simulink model "Catwell_Rom"  (R2023b)
settings: Solver=FixedStepDiscrete  StartTime=0.0  StopTime=3.999  FixedStep=0.02  RelTol=1e-3
libraries: Pathfinding_lib x2, drivinglib x1, SignalEditorBlockLib x1, matrix_library x1
settings Model: Creator=FIRSTMentor  LastModifiedBy=FIRSTMentor
settings OptimizationCC: DefaultParameterBehavior=Inlined  EnhancedBackFolding=on  PassReuseOutputArgsAs=Individual arguments  ZeroExternalMemoryAtStartup=off  ZeroInternalMemoryAtStartup=off  OptimizeBlockOrder=speed  DifferentSizesBufferReuse=on  OptimizationCustomize=off  EfficientTunableParamExpr=on
settings DebuggingCC: ParameterTunabilityLossMsg=error
settings SFSimCC: MATLABDynamicMemAlloc=off
settings RTWCC: Description=Embedded Coder  SystemTargetFile=ert.tlc  GenCodeOnly=on  TemplateMakefile=ert_default_tmf  Toolchain=Microsoft Visual C++ 2022 v17.0 | CMake/nmake (64-bit Windows)  BuildConfiguration=Release
settings CodeAppCC: ForceParamTrailComments=on  IgnoreCustomStorageClasses=off  OperatorAnnotations=on  SimulinkDataObjDesc=on  SFDataObjDesc=on  InsertBlockDesc=on
settings ERTTargetCC: TargetLangStandard=C99 (ISO)  GenerateSampleERTMain=on  InlinedParameterPlacement=NonHierarchical  ERTCustomFileTemplate=example_file_process.tlc

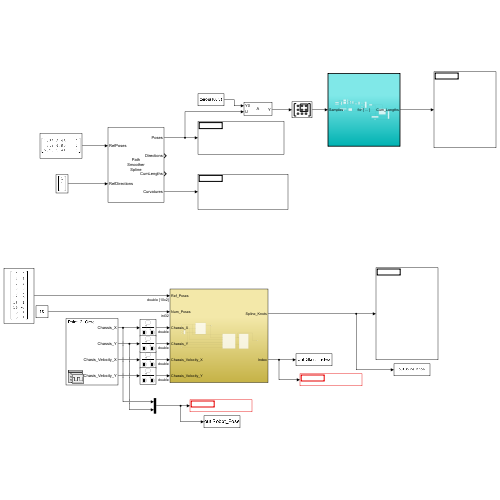
[thumbnail: Simulink's stored preview of the top-level diagram]
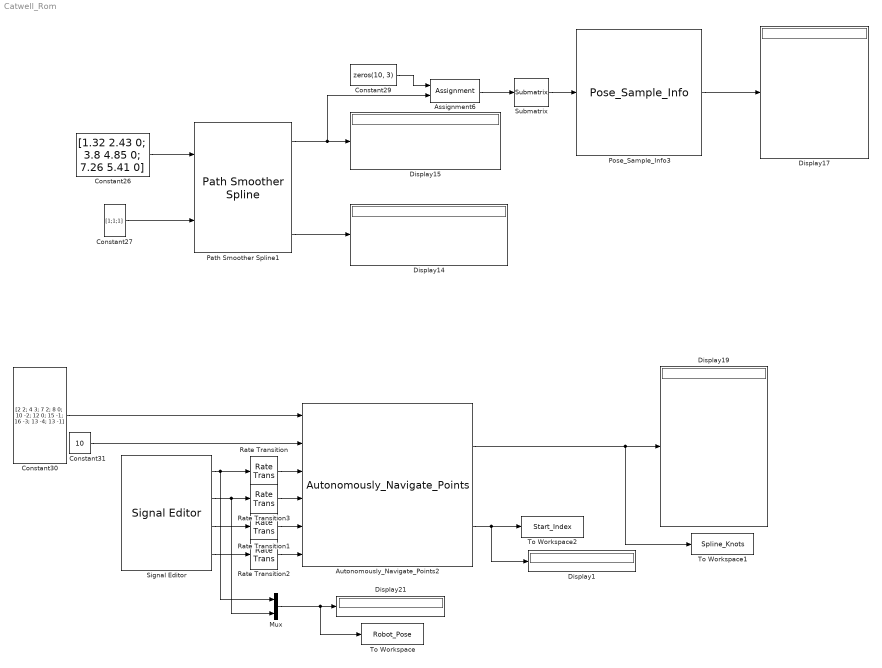
== system Catwell_Rom ==
  Assignment6 : Assignment  NumberOfDimensions=2  DiagnosticForDimensions=Warning  IndexOptions=Starting index (dialog),Starting index (dialog)  Indices=1,1  OutputSizes=1,1
  Autonomously_Navigate_Points2 : Pathfinding_lib/Autonomously_Navigate_Points  SystemSampleTime=-1  VariantActivationTime=update diagram  AllowFlexibleInterface=on  Latency=0  AutoFrameSizeCalculation=off
  Constant26 : Constant  Value=[1.32 2.43 0; 3.8 4.85 0; 7.26 5.41 0]  VectorParams1D=off
  Constant27 : Constant  Value=[1;1;1]  VectorParams1D=off
  Constant29 : Constant  Value=zeros(10, 3)
  Constant30 : Constant  Value=[2 2; 4 3; 7 2; 8 0; 10 -2; 12 0; 15 -1; 16 -3; 13 -4; 13 -1]
  Constant31 : Constant  Value=10  OutDataTypeStr=int32
  Display{1,14..15,17,19,21} (6 alike) : Display
  Mux : Mux  Inputs=2
  Path Smoother Spline1 : drivinglib/Path Smoother Spline  NumSmoothPoses=10  MinSeparation=1e-3  SampleTime=0.5  ShowOptionalOutports=on  SimulateUsing=Code generation
  Pose_Sample_Info3 : Pathfinding_lib/Pose_Sample_Info  SystemSampleTime=-1  VariantActivationTime=update diagram  AllowFlexibleInterface=on  Latency=0  AutoFrameSizeCalculation=off
  Rate Transition{,1..3} (4 alike) : RateTransition  OutPortSampleTime=t_sample
  Signal Editor : SignalEditorBlockLib/Signal Editor  FileName=Catwell_Rom_Path_Test_Cases.mat  ActiveScenario=Point_2_Circle  ActiveSignal=Chassis_X  IsBus=off  OutputBusObjectStr=Bus: BusObject  SampleTime=0  Interpolate=off  ZeroCross=off  OutputAfterFinalValue=Setting to zero  Unit=inherit  PreserveSignalName=on  ApplySigPropsToAllScenarios=on  ApplySigPropsToAllSignals=off
  Submatrix : matrix_library/Submatrix  RowSpan=All rows  RowStartMode=First  RowStartIndex=1  RowEndMode=Last  RowEndIndex=1  ColSpan=Range of columns  ColStartMode=First  ColStartIndex=1  ColEndMode=Offset from last  ColEndIndex=1
  To Workspace : ToWorkspace  VariableName=Robot_Pose  SampleTime=-1
      settings: Save2DSignal=2-D array (concatenate along first dimension)
  To Workspace1 : ToWorkspace  VariableName=Spline_Knots  SampleTime=-1
  To Workspace2 : ToWorkspace  VariableName=Start_Index  SampleTime=-1
  wires:
  Constant26/1 -> Path Smoother Spline1/1
  Constant27/1 -> Path Smoother Spline1/2
  Path Smoother Spline1/4 -> Display14/1
  Path Smoother Spline1/1 -> Assignment6/2, Display15/1
  Submatrix/1 -> Pose_Sample_Info3/1
  Pose_Sample_Info3/1 -> Display17/1
  Constant29/1 -> Assignment6/1
  Assignment6/1 -> Submatrix/1
  Constant30/1 -> Autonomously_Navigate_Points2/1
  Constant31/1 -> Autonomously_Navigate_Points2/2
  Autonomously_Navigate_Points2/1 -> To Workspace1/1, Display19/1
  Signal Editor/1 -> Mux/1, Rate Transition/1
  Signal Editor/2 -> Mux/2, Rate Transition3/1
  Signal Editor/3 -> Rate Transition1/1
  Signal Editor/4 -> Rate Transition2/1
  Rate Transition/1 -> Autonomously_Navigate_Points2/3
  Rate Transition1/1 -> Autonomously_Navigate_Points2/5
  Rate Transition2/1 -> Autonomously_Navigate_Points2/6
  Rate Transition3/1 -> Autonomously_Navigate_Points2/4
  Mux/1 -> To Workspace/1, Display21/1
  Autonomously_Navigate_Points2/2 -> Display1/1, To Workspace2/1
